simulink model "MathmeticalModaling"  (R2023a)
settings: Solver=VariableStepAuto  StartTime=0.0  StopTime=10.0  RelTol=1e-3
settings Model: Creator=Hp  LastModifiedBy=Hp

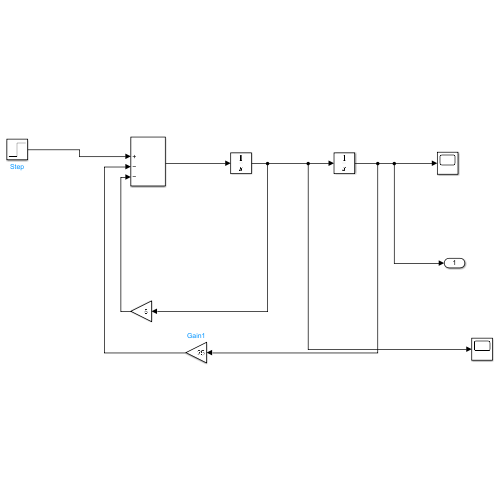
[thumbnail: Simulink's stored preview of the top-level diagram]
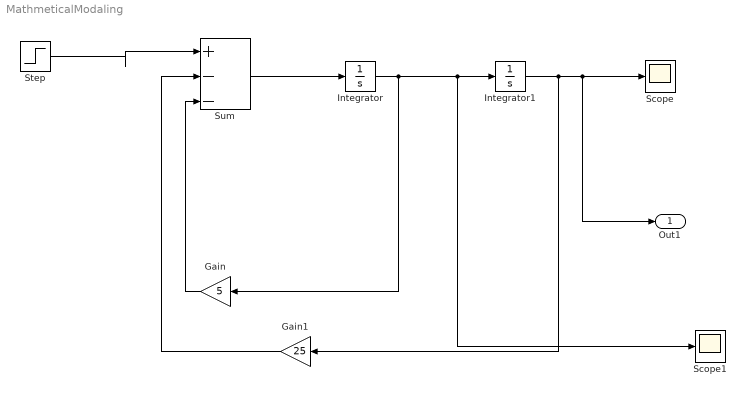
== system MathmeticalModaling ==
  Gain : Gain  Gain=5
  Gain1 : Gain  Gain=25
  Integrator : Integrator
  Integrator1 : Integrator
  Scope : Scope
  Scope1 : Scope
  Step : Step  After=25  SampleTime=0
  Sum : Sum  Inputs=|+--
  Out1 : Outport
  wires:
  Integrator/1 -> Gain/1, Scope1/1, Integrator1/1
  Integrator1/1 -> Gain1/1, Out1/1, Scope/1
  Gain/1 -> Sum/3
  Sum/1 -> Integrator/1
  Gain1/1 -> Sum/2
  Step/1 -> Sum/1
